simulink model "dart_model"  (R2023b)
settings: Solver=VariableStepAuto  StartTime=0.0  StopTime=10  FixedStep=0.0005  RelTol=1e-3  AbsTol=1e-3  EnableMultiTasking=on
values from neighbouring files (symbols this model uses):
  Param_Mus_MEE = Library_mtu_simulink_mtu_standard_parameters(Param_Mus_MEE)    [init_muscle_MEE.m]
  Param_Mus_MEF = Library_mtu_simulink_mtu_standard_parameters(Param_Mus_MEF)    [init_muscle_MEF.m]
undefined symbols (not defined in the file or in its folder): X, Y, Z
libraries: sm_lib x43, nesl_utility x10, Library_mtu_simulink x4, simulink x1
(part 2 of 2)

== matlab function dart_model/MATLAB Function ==
  data: u input; y output
function y = tanh(u)

y = 0.4*tanh(0.5*u-2)-tanh(-2)*0.4+0.01;

== matlab function dart_model/MATLAB Function1 ==
  data: u input; y output
function y = minus_tanh(u)

y = -0.4*tanh(0.5*u)+0.4;
